simulink model "simulation_test"  (R2021a)
settings: Solver=FixedStepDiscrete  StartTime=0.0  StopTime=400.0  FixedStep=1  RelTol=1e-3
libraries: xbsIndex_r4 x4, hdlsllib x1, xps_library x1, dspsrcs4 x1
(part 3 of 3)

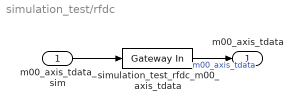
== system simulation_test/rfdc ==
  m00_axis_tdata_sim : Inport
  simulation_test_rfdc_m00_axis_tdata : xbsIndex_r4/Gateway In  gui_display_data_type=Fixed-point  arith_type="Signed  (2's comp)"  n_bits=128  bin_pt=0  preci_type=Single  exp_width=8  frac_width=24  rows=1  columns=1  quantization="Round  (unbiased: +/- Inf)"  overflow=Saturate  period=1  UseAsADC=off  ADCChannel='1'  interface=None  automatic_assignment=on  address_offset=hex2dec('00')  intf_name=''  intf_description=''  default_value=0  timing_constraint=None  locs_specified=off  LOCs={}  io_standard={}  inherit_from_input=off  hdl_port=on  dbl_ovrd=off  block_type=gatewayin
  m00_axis_tdata : Outport
  wires:
  m00_axis_tdata_sim/1 -> simulation_test_rfdc_m00_axis_tdata/1
  simulation_test_rfdc_m00_axis_tdata/1 -> m00_axis_tdata/1  "m00_axis_tdata"
